simulink model "productionLineS"  (R2025a)
settings: Solver=VariableStepAuto  StartTime=0.0  StopTime=10.0  RelTol=1e-3
libraries: NSA_DEVS_SINKS x12, ProductionLineLib_CM x7, NSA_DEVS_SOURCES x2, NSA_DEVS_LOGISTICS x1
settings Model: Creator=peter  LastModifiedBy=peter
settings RTWCC: GPUComputeCapability=3.5

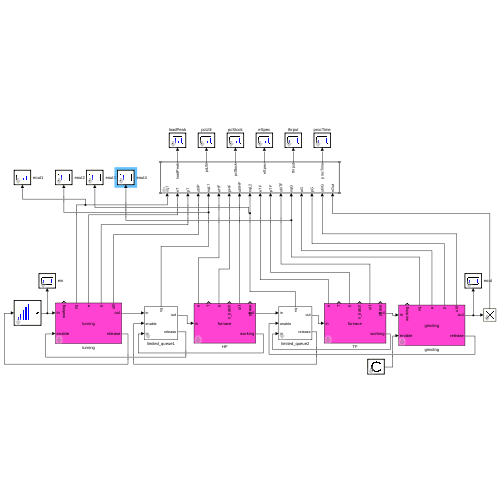
[thumbnail: Simulink's stored preview of the top-level diagram]
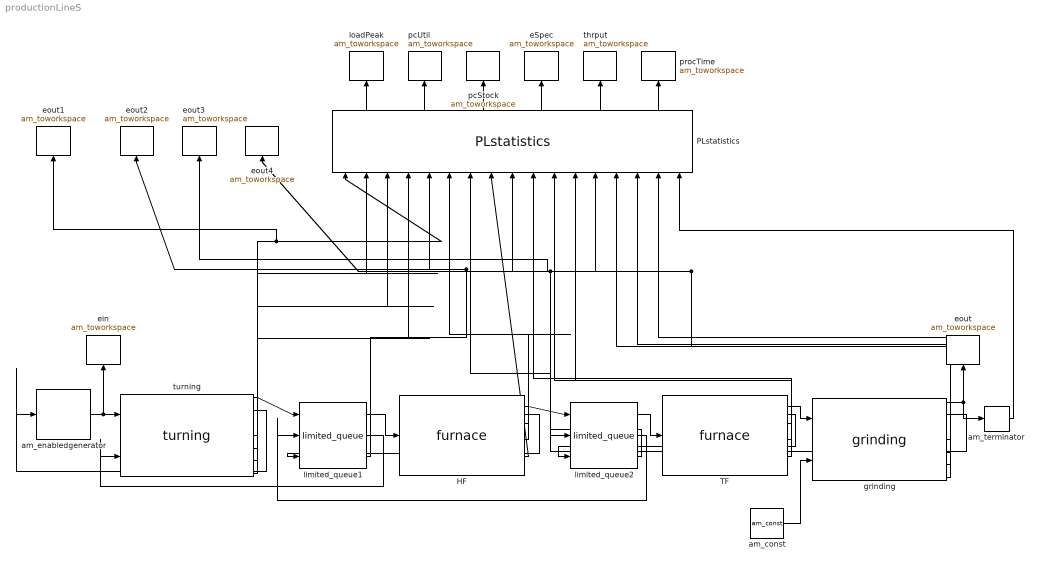
== system productionLineS ==
  HF : ProductionLineLib_CM/furnace  PH=20000  Co=12000  k_A=10  Te=25  P0=2000  P_unload=120000  holding_time=180*3  Tsoll=800  Kapa=15  tauInt=[0,1]  tauCont=[0,1]  tau=[0,1]  debug=0
      link override unbatch: tau=[0,1]  tD=[0,2]
  PLstatistics : ProductionLineLib_CM/PLstatistics  tau=[0,1]  debug=0
  TF : ProductionLineLib_CM/furnace  PH=20000  Co=12000  k_A=10  Te=25  P0=2000  P_unload=50000  holding_time=360*3  Tsoll=400  Kapa=15  tauInt=[0,1]  tauCont=[0,1]  tau=[0,1]  debug=0
      link override unbatch: tau=[0,1]  tD=[0,6]
  am_const : NSA_DEVS_SOURCES/am_const  value=true  sendTime=[0,1]  debug=0
      settings: SourceProductName=Sources
  am_enabledgenerator : NSA_DEVS_SOURCES/am_enabledgenerator  tG=20  n0=1  nG=50  tD=[0,2]  tau=[0,1]  debug=0
      settings: SourceProductName=Sources
  am_terminator : NSA_DEVS_LOGISTICS/am_terminator  countyEmptyInputs=false  tau_copy=[0,1]  debug_copy=0
      settings: SourceProductName=Logistics
  eSpec : NSA_DEVS_SINKS/am_toworkspace  varname="\"eSpec\""  t0=0  format="\"vector\""  tau=[0,5]  debug=0
      settings: SourceProductName=Sinks
  ein : NSA_DEVS_SINKS/am_toworkspace  varname="\"eIn\""  t0=0  format="\"vector\""  tau=[0,5]  debug=0
      settings: SourceProductName=Sinks
  eout : NSA_DEVS_SINKS/am_toworkspace  varname="\"eOut\""  t0=0  format="\"vector\""  tau=[0,0.5]  debug=0
      settings: SourceProductName=Sinks
  eout1 : NSA_DEVS_SINKS/am_toworkspace  varname="\"test1\""  t0=0  format="\"vector\""  tau=[0,0.5]  debug=0
      settings: SourceProductName=Sinks
  eout2 : NSA_DEVS_SINKS/am_toworkspace  varname="\"test2\""  t0=0  format="\"vector\""  tau=[0,0.5]  debug=0
      settings: SourceProductName=Sinks
  eout3 : NSA_DEVS_SINKS/am_toworkspace  varname="\"test3\""  t0=0  format="\"vector\""  tau=[0,0.5]  debug=0
      settings: SourceProductName=Sinks
  eout4 : NSA_DEVS_SINKS/am_toworkspace  varname="\"test4\""  t0=0  format="\"vector\""  tau=[0,0.5]  debug=0
      settings: SourceProductName=Sinks
  grinding : ProductionLineLib_CM/grinding  vfr1=0.48  vfr2=0.19  vfr3=0.03  vc=30  max_fifo=400  grinding_time=3*60  tauInt=[0,1]  tauCont=[0,1]  tau=[0,1]  debug=0
      link override combine3: tD=[0,2]
      link override input_queue: tau=[0,1]  tD=[0,2]
      link override input_queue/distribute3: tau=[0,1]
  limited_queue1 : ProductionLineLib_CM/limited_queue  max_fifo=400  tD=[0,2]  tau=[0,1]  debug=0
  limited_queue2 : ProductionLineLib_CM/limited_queue  max_fifo=400  tD=[0,2]  tau=[0,1]  debug=0
  loadPeak : NSA_DEVS_SINKS/am_toworkspace  varname="\"loadPeak\""  t0=0  format="\"vector\""  tau=[0,5]  debug=0
      settings: SourceProductName=Sinks
  pcStock : NSA_DEVS_SINKS/am_toworkspace  varname="\"pcStock\""  t0=0  format="\"vector\""  tau=[0,5]  debug=0
      settings: SourceProductName=Sinks
  pcUtil : NSA_DEVS_SINKS/am_toworkspace  varname="\"pcUtil\""  t0=0  format="\"vector\""  tau=[0,5]  debug=0
      settings: SourceProductName=Sinks
  procTime : NSA_DEVS_SINKS/am_toworkspace  varname="\"procTime\""  t0=0  format="\"vector\""  tau=[0,5]  debug=0
      settings: SourceProductName=Sinks
  thrput : NSA_DEVS_SINKS/am_toworkspace  varname="\"thrput\""  t0=0  format="\"vector\""  tau=[0,5]  debug=0
      settings: SourceProductName=Sinks
  turning : ProductionLineLib_CM/turning  ap=0.5  f=0.1  vc=150  max_fifo=400  turning_time=2*60  tauInt=[0,1]  tauCont=[0,1]  tau=[0,1]  debug=0
      link override combine3: tD=[0,2]
      link override input_queue: tau=[0,1]  tD=[0,2]
      link override input_queue/distribute3: tau=[0,1]
  wires:
  am_enabledgenerator/1 -> ein/1, turning/1
  turning/1 -> limited_queue1/1
  limited_queue1/1 -> HF/1
  HF/1 -> limited_queue2/1
  limited_queue2/1 -> TF/1
  TF/1 -> grinding/1
  grinding/1 -> eout/1, am_terminator/1
  limited_queue1/2 -> turning/2
  limited_queue2/2 -> limited_queue1/2
  HF/2 -> limited_queue1/3
  grinding/2 -> limited_queue2/2
  TF/2 -> limited_queue2/3
  am_const/1 -> grinding/2
  turning/4 -> eout1/1, PLstatistics/1
  turning/5 -> PLstatistics/2
  turning/6 -> PLstatistics/3
  turning/7 -> PLstatistics/4
  am_terminator/1 -> PLstatistics/17
  PLstatistics/1 -> loadPeak/1
  PLstatistics/2 -> pcUtil/1
  PLstatistics/3 -> pcStock/1
  PLstatistics/4 -> eSpec/1
  limited_queue1/3 -> eout2/1, PLstatistics/5
  HF/3 -> PLstatistics/6
  HF/5 -> PLstatistics/7
  HF/7 -> PLstatistics/8
  limited_queue2/3 -> eout3/1, PLstatistics/9
  TF/3 -> PLstatistics/10
  TF/5 -> PLstatistics/11
  TF/7 -> PLstatistics/12
  grinding/4 -> eout4/1, PLstatistics/13
  grinding/5 -> PLstatistics/14
  grinding/6 -> PLstatistics/15
  grinding/7 -> PLstatistics/16
  PLstatistics/5 -> thrput/1
  PLstatistics/6 -> procTime/1
  turning/2 -> am_enabledgenerator/1
